simulink model "my_controller"  (R2020a)
settings: Solver=VariableStepAuto  StartTime=0.0  StopTime=1  RelTol=1e-3
libraries: simulink_extras x2, fuzblock x1
settings Model: Creator=IamAM  LastModifiedBy=IamAM

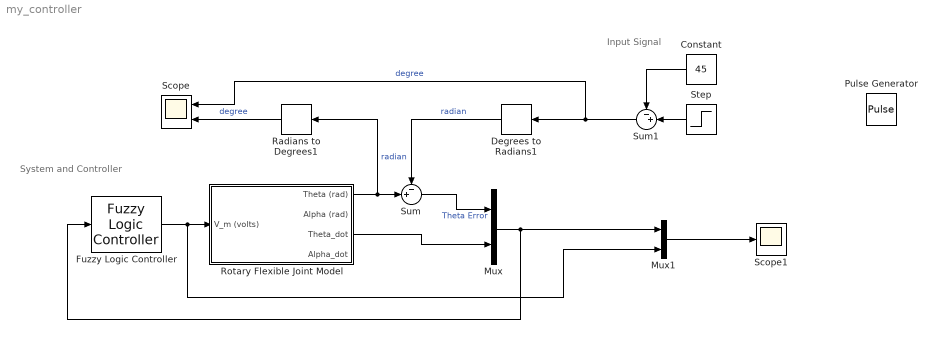
== system my_controller ==
  note: System and Controller
  note: Input Signal
  Constant : Constant  Value=45
  Degrees to Radians1 : simulink_extras/Transformations/Degrees to Radians
  Fuzzy Logic Controller : fuzblock/Fuzzy Logic  Controller  FIS='my_fis.fis'  OutputSampleNumber=101  DataType=double  FuzzifiedInputs=off  RuleFiringStrengths=off  RuleOutputs=off  AggregatedOutputs=off  SimulateUsing=Interpreted execution  OutOfRangeInputValueMessage=warning  NoRuleFiredMessage=warning  EmptyOutputFuzzySetMessage=warning
  Mux : Mux  Inputs=2
  Mux1 : Mux  Inputs=2
  Pulse Generator : DiscretePulseGenerator  PulseType=Time based  Amplitude=90  Period=3  PulseWidth=50
  Radians to Degrees1 : simulink_extras/Transformations/Radians to Degrees
  Rotary Flexible Joint Model : Subsystem
  Scope : Scope  NumInputPorts=2
  Scope1 : Scope
  Step : Step  Time=0.01  After=90  SampleTime=0
  Sum : Sum  Inputs=-+|
  Sum1 : Sum  Inputs=-+|
  wires:
  Degrees to Radians1/1 -> Sum/1  "radian"
  Radians to Degrees1/1 -> Scope/2  "degree"
  Constant/1 -> Sum1/1
  Sum/1 -> Mux/1  "Theta Error"
  Mux/1 -> Mux1/1, Fuzzy Logic Controller/1
  Sum1/1 -> Degrees to Radians1/1, Scope/1  "degree"
  Step/1 -> Sum1/2
  Fuzzy Logic Controller/1 -> Mux1/2, Rotary Flexible Joint Model/1(V_m (volts))
  Rotary Flexible Joint Model/1(Theta (rad)) -> Radians to Degrees1/1, Sum/2  "radian"
  Mux1/1 -> Scope1/1
  Rotary Flexible Joint Model/3(Theta_dot) -> Mux/2

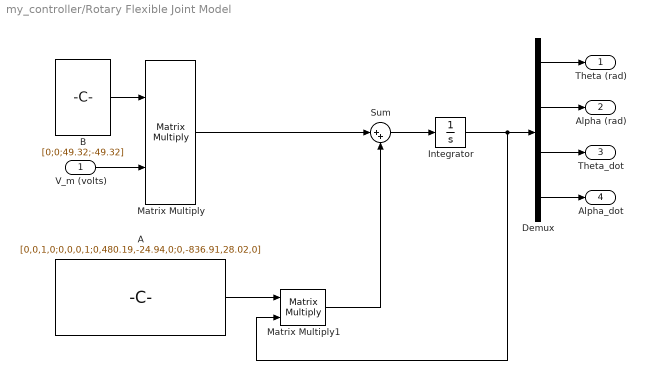
== system my_controller/Rotary Flexible Joint Model ==
  V_m (volts) : Inport
  A : Constant  Value=[0,0,1,0;0,0,0,1;0,480.19,-24.94,0;0,-836.91,28.02,0]
  B : Constant  Value=[0;0;49.32;-49.32]  VectorParams1D=off
  Demux : Demux
  Integrator : Integrator
  Matrix Multiply : Product  Multiplication=Matrix(*)
  Matrix Multiply1 : Product  Multiplication=Matrix(*)
  Sum : Sum  Inputs=|++
  Theta (rad) : Outport
  Alpha (rad) : Outport  Port=2
  Theta_dot : Outport  Port=3
  Alpha_dot : Outport  Port=4
  wires:
  V_m (volts)/1 -> Matrix Multiply/2
  B/1 -> Matrix Multiply/1
  A/1 -> Matrix Multiply1/1
  Matrix Multiply1/1 -> Sum/2
  Matrix Multiply/1 -> Sum/1
  Sum/1 -> Integrator/1
  Integrator/1 -> Matrix Multiply1/2, Demux/1
  Demux/1 -> Theta (rad)/1
  Demux/2 -> Alpha (rad)/1
  Demux/3 -> Theta_dot/1
  Demux/4 -> Alpha_dot/1
